simulink model "Integration_HILS_Filtered"  (R2023b)
settings: Solver=FixedStepAuto  StartTime=0.0  StopTime=inf  FixedStep=0.01  RelTol=1e-3  EnableMultiTasking=on
values from neighbouring files (symbols this model uses):
  batteryChargeRate = 0.0005    [paraHILS_File.m]
  batteryUpdateTime = 0.1    [paraHILS_File.m]
  batteryUseRate = 0.01    [paraHILS_File.m]
  encoder_scale = 1/12/4    (= 0.0208333333333)    [paraHILS_File.m]
  EncoderCutOffFreq = 48.1    [paraHILS_File.m]
  Ki = 10.0    (= 10)    [paraHILS_File.m]
  Kp = 10.0    (= 10)    [paraHILS_File.m]
  LimitMotorSpd = 0.8    [paraHILS_File.m]
  oilChargeRate = 2    [paraHILS_File.m]
  oilUpdateTime = 0.1    [paraHILS_File.m]
  oilUseRate = 0.01    [paraHILS_File.m]
  Vlim = 12    [paraHILS_File.m]
undefined symbols (not defined in the file or in its folder): MapVarRes2RPS
libraries: arduinolib x17, arduinosensorlib x2, simulink x2, cstblocks x2, dspstat3 x1
settings Model: ExtModeTrigDuration=2  Creator=sein  LastModifiedBy=hangbe
settings OptimizationCC: EnhancedBackFolding=on  PassReuseOutputArgsAs=Individual arguments  ZeroExternalMemoryAtStartup=off  ZeroInternalMemoryAtStartup=off  MaxStackSize=64  OptimizeBlockOrder=speed  DifferentSizesBufferReuse=on  OptimizationCustomize=off  EfficientTunableParamExpr=on
settings DebuggingCC: ParameterTunabilityLossMsg=error
settings HardwareCC: ProdBitPerInt=16  ProdBitPerPointer=16  ProdBitPerSizeT=16  ProdBitPerPtrDiffT=16  ProdLargestAtomicFloat=None  ProdWordSize=8  ProdHWDeviceType=Atmel->AVR
settings SFSimCC: MATLABDynamicMemAlloc=off
settings RTWCC: Description=Embedded Coder  SystemTargetFile=ert.tlc  HardwareBoard=Arduino Mega 2560  TemplateMakefile=ert_default_tmf  Toolchain=Arduino AVR  BuildConfiguration=Faster Runs
settings CodeAppCC: ForceParamTrailComments=on  IgnoreCustomStorageClasses=off  OperatorAnnotations=on  SimulinkDataObjDesc=on  SFDataObjDesc=on  InsertBlockDesc=on
settings ERTTargetCC: SupportContinuousTime=on  SupportVariableSizeSignals=on  ExtModeTransport=3  ExtModeStaticAlloc=on  ExtModeAutomaticAllocSize=off  ExtModeStaticAllocSize=2048  ExtModeMexFile=ext_xcp  ExtModeIntrfLevel=Level2 - Open

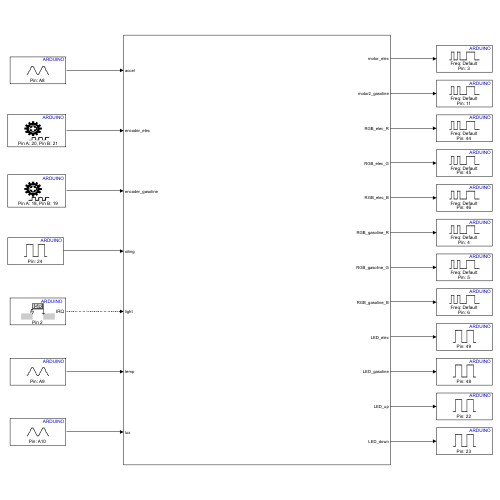
[thumbnail: Simulink's stored preview of the top-level diagram]
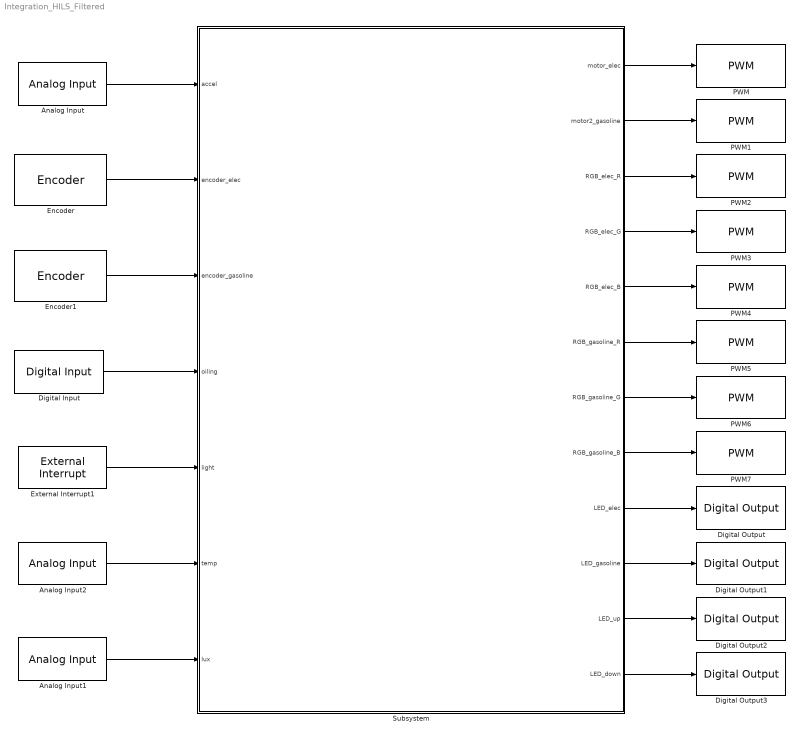
== system Integration_HILS_Filtered ==
  Analog Input : arduinolib/Analog Input  pinNumber=8  ReadResultsOnly=off  ConversionTriggerSource=Software  ExternalTriggerType=uint32( 0 )  OutputDataType=uint16  EnableConversionCompleteNotify=off  EnableOuputStatus=off  SampleTime=-1  blockPlatform=arduino
  Analog Input1 : arduinolib/Analog Input  pinNumber=10  ReadResultsOnly=off  ConversionTriggerSource=Software  ExternalTriggerType=uint32( 0 )  OutputDataType=uint16  EnableConversionCompleteNotify=off  EnableOuputStatus=off  SampleTime=-1  blockPlatform=arduino
  Analog Input2 : arduinolib/Analog Input  pinNumber=9  ReadResultsOnly=off  ConversionTriggerSource=Software  ExternalTriggerType=uint32( 0 )  OutputDataType=uint16  EnableConversionCompleteNotify=off  EnableOuputStatus=off  SampleTime=-1  blockPlatform=arduino
  Digital Input : arduinolib/Digital Input  pinNumber=24  mode=Default  Direction=input  SampleTime=0.1  blockPlatform=arduino
  Digital Output : arduinolib/Digital Output  pinNumber=49  Direction=output  blockPlatform=arduino
  Digital Output1 : arduinolib/Digital Output  pinNumber=48  Direction=output  blockPlatform=arduino
  Digital Output2 : arduinolib/Digital Output  pinNumber=22  Direction=output  blockPlatform=arduino
  Digital Output3 : arduinolib/Digital Output  pinNumber=23  Direction=output  blockPlatform=arduino
  Encoder : arduinosensorlib/Encoder  InputA=20  InputB=21  Mode=No reset  SampleTime=-1
  Encoder1 : arduinosensorlib/Encoder  InputA=18  InputB=19  Mode=No reset  SampleTime=-1
  External Interrupt1 : arduinolib/External Interrupt  Pin=2  PullUp=off  Mode=RISING  InterruptSimulationInput=off
  PWM : arduinolib/PWM  pinNumber=3  frequencyType=Default  desiredFrequency=490.2  achievableFrequency=490.2
  PWM1 : arduinolib/PWM  pinNumber=11  frequencyType=Default  desiredFrequency=490.2  achievableFrequency=490.2
  PWM2 : arduinolib/PWM  pinNumber=44  frequencyType=Default  desiredFrequency=490.2  achievableFrequency=490.2
  PWM3 : arduinolib/PWM  pinNumber=45  frequencyType=Default  desiredFrequency=490.2  achievableFrequency=490.2
  PWM4 : arduinolib/PWM  pinNumber=46  frequencyType=Default  desiredFrequency=490.2  achievableFrequency=490.2
  PWM5 : arduinolib/PWM  pinNumber=4  frequencyType=Default  desiredFrequency=490.2  achievableFrequency=490.2
  PWM6 : arduinolib/PWM  pinNumber=5  frequencyType=Default  desiredFrequency=490.2  achievableFrequency=490.2
  PWM7 : arduinolib/PWM  pinNumber=6  frequencyType=Default  desiredFrequency=490.2  achievableFrequency=490.2
  Subsystem : Subsystem
  wires:
  Analog Input/1 -> Subsystem/1(accel)
  Encoder/1 -> Subsystem/2(encoder_elec)
  Digital Input/1 -> Subsystem/4(oiling)
  External Interrupt1/1 -> Subsystem/5(light)
  Analog Input2/1 -> Subsystem/6(temp)
  Analog Input1/1 -> Subsystem/7(lux)
  Subsystem/1(motor_elec) -> PWM/1
  Subsystem/2(motor2_gasoline) -> PWM1/1
  Subsystem/3(RGB_elec_R) -> PWM2/1
  Subsystem/4(RGB_elec_G) -> PWM3/1
  Subsystem/5(RGB_elec_B) -> PWM4/1
  Subsystem/6(RGB_gasoline_R) -> PWM5/1
  Subsystem/7(RGB_gasoline_G) -> PWM6/1
  Subsystem/8(RGB_gasoline_B) -> PWM7/1
  Subsystem/9(LED_elec) -> Digital Output/1
  Subsystem/10(LED_gasoline) -> Digital Output1/1
  Subsystem/11(LED_up) -> Digital Output2/1
  Subsystem/12(LED_down) -> Digital Output3/1
  Encoder1/1 -> Subsystem/3(encoder_gasoline)

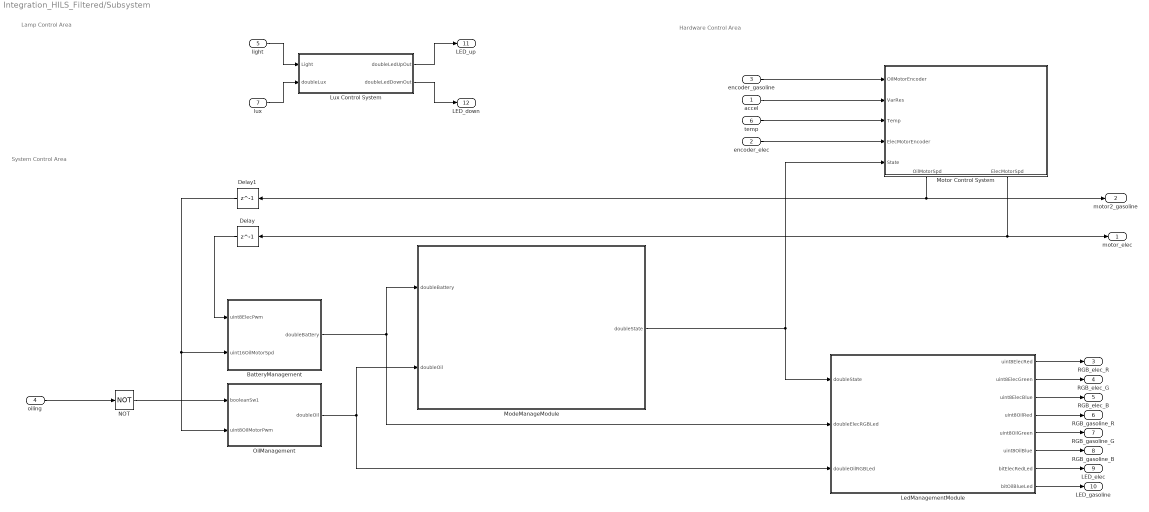
== system Integration_HILS_Filtered/Subsystem ==
  note: Lamp Control Area
  note: Hardware Control Area
  note: System Control Area
  accel : Inport
  encoder_elec : Inport  Port=2
  encoder_gasoline : Inport  Port=3
  oiling : Inport  Port=4
  light : Inport  Port=5
  temp : Inport  Port=6
  lux : Inport  Port=7
  BatteryManagement : Subsystem
  Delay : Delay  DelayLength=1
  Delay1 : Delay  DelayLength=1
  LedManagementModule : Subsystem
  Lux Control System : Subsystem
  ModeManageModule : Subsystem
  Motor Control System : Subsystem
      settings: PortSchema="{\"entries\":[{\"content\":{\"sides\":[{\"content\":{\"connectorIds\":[\"In1\",\"In2\",\"In3\",\"In4\",\"In5\"]},\"type\":\"ConnectorPlacement.EquallySpacedRectSide\",\"uuid\":\"d78dbdb5-4c64-485d-9b60-ddf3d4c9e050\"},{\"content\":{\"side\":\"RIGHT\"},\"type\":\"ConnectorPlacement.EquallySpacedRectSide\",\"uuid\":\"e4947276-b3db-4eab-ab89-2db109b5b76f\"},{\"content\":{\"side\":\"TOP\"},\"type\":\"ConnectorPlacement.EquallySpacedRectSide\",\"uuid\":\"f10de6be-2a9c-4a01-854d-c691ec39bdb2\"},{\"content\":{\"connectorIds\":[\"Out1\",\"Out2\"],\"side\":\"BOTTOM\"},\"type\":\"ConnectorPlacement.EquallySpacedRectSide\",\"uuid\":\"8b2dfeae-af3a-4cb1-8e5d-8c4928cafd33\"}]},\"type\":\"ConnectorPlacement.EquallySpacedConnector\",\"uuid\":\"966cd9e0-5a43-41a6-af76-62067303310a\"}],\"packageUris\":[\"http://schema.mathworks.com/mf0/Connector/R2020b\"],\"version\":\"1.0\"}"
  NOT : Logic  Operator=NOT  IconShape=distinctive  AllPortsSameDT=off  OutDataTypeStr=boolean
  OilManagement : Subsystem
  motor_elec : Outport
  motor2_gasoline : Outport  Port=2
  RGB_elec_R : Outport  Port=3
  RGB_elec_G : Outport  Port=4
  RGB_elec_B : Outport  Port=5
  RGB_gasoline_R : Outport  Port=6
  RGB_gasoline_G : Outport  Port=7
  RGB_gasoline_B : Outport  Port=8
  LED_elec : Outport  Port=9
  LED_gasoline : Outport  Port=10
  LED_up : Outport  Port=11
  LED_down : Outport  Port=12
  wires:
  LedManagementModule/1(uint8ElecRed) -> RGB_elec_R/1
  LedManagementModule/2(uint8ElecGreen) -> RGB_elec_G/1
  LedManagementModule/3(uint8ElecBlue) -> RGB_elec_B/1
  LedManagementModule/4(uint8OilRed) -> RGB_gasoline_R/1
  LedManagementModule/5(uint8OilGreen) -> RGB_gasoline_G/1
  LedManagementModule/6(uint8OilBlue) -> RGB_gasoline_B/1
  LedManagementModule/7(bitElecRedLed) -> LED_elec/1
  LedManagementModule/8(bitOilBlueLed) -> LED_gasoline/1
  ModeManageModule/1(doubleState) -> Motor Control System/5(State), LedManagementModule/1(doubleState)
  OilManagement/1(doubleOil) -> LedManagementModule/3(doubleOilRGBLed), ModeManageModule/2(doubleOil)
  oiling/1 -> NOT/1
  Delay/1 -> BatteryManagement/1(uint8ElecPwm)
  Delay1/1 -> OilManagement/2(uint8OilMotorPwm), BatteryManagement/2(uint16OilMotorSpd)
  NOT/1 -> OilManagement/1(booleanSw1)
  BatteryManagement/1(doubleBattery) -> LedManagementModule/2(doubleElecRGBLed), ModeManageModule/1(doubleBattery)
  light/1 -> Lux Control System/1(Light)
  lux/1 -> Lux Control System/2(doubleLux)
  Lux Control System/1(doubleLedUpOut) -> LED_up/1
  Lux Control System/2(doubleLedDownOut) -> LED_down/1
  Motor Control System/2(ElecMotorSpd) -> motor_elec/1, Delay/1
  Motor Control System/1(OilMotorSpd) -> motor2_gasoline/1, Delay1/1
  encoder_gasoline/1 -> Motor Control System/1(OilMotorEncoder)
  accel/1 -> Motor Control System/2(VarRes)
  temp/1 -> Motor Control System/3(Temp)
  encoder_elec/1 -> Motor Control System/4(ElecMotorEncoder)

== system Integration_HILS_Filtered/Subsystem/BatteryManagement ==
  uint8ElecPwm : Inport
  uint16OilMotorSpd : Inport  Port=2
  Chart : Stateflow chart  TreatAsAtomicUnit=on
  Data Type Conversion : DataTypeConversion  OutDataTypeStr=double  SaturateOnIntegerOverflow=off  RndMeth=Floor
  Data Type Conversion1 : DataTypeConversion  OutDataTypeStr=double  SaturateOnIntegerOverflow=off  RndMeth=Floor
  Display : Display
  doubleBattery : Outport  OutDataTypeStr=double
  wires:
  uint8ElecPwm/1 -> Data Type Conversion/1
  Chart/1(uint8Battery) -> doubleBattery/1, Display/1
  uint16OilMotorSpd/1 -> Data Type Conversion1/1
  Data Type Conversion/1 -> Chart/1(uint8ElecPwm)
  Data Type Conversion1/1 -> Chart/2(uint16OilMotorSpd)

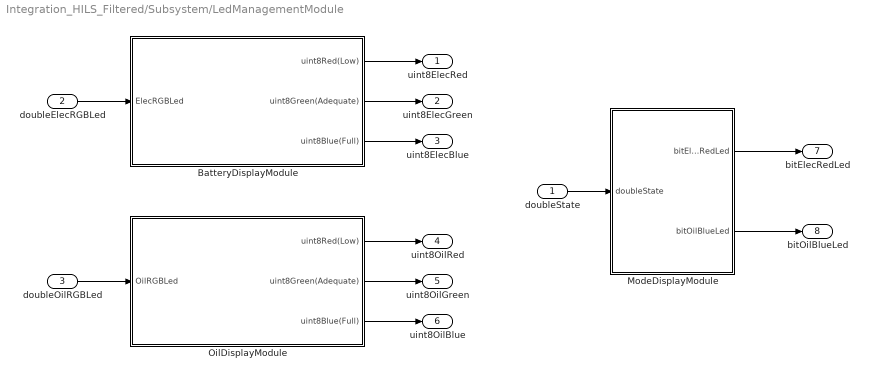
== system Integration_HILS_Filtered/Subsystem/LedManagementModule ==
  doubleState : Inport
  doubleElecRGBLed : Inport  Port=2
  doubleOilRGBLed : Inport  Port=3
  BatteryDisplayModule : Subsystem
  ModeDisplayModule : Subsystem
  OilDisplayModule : Subsystem
  uint8ElecRed : Outport
  uint8ElecGreen : Outport  Port=2
  uint8ElecBlue : Outport  Port=3
  uint8OilRed : Outport  Port=4
  uint8OilGreen : Outport  Port=5
  uint8OilBlue : Outport  Port=6
  bitElecRedLed : Outport  Port=7
  bitOilBlueLed : Outport  Port=8
  wires:
  OilDisplayModule/2(uint8Green(Adequate)) -> uint8OilGreen/1
  OilDisplayModule/3(uint8Blue(Full)) -> uint8OilBlue/1
  BatteryDisplayModule/1(uint8Red(Low)) -> uint8ElecRed/1
  BatteryDisplayModule/2(uint8Green(Adequate)) -> uint8ElecGreen/1
  OilDisplayModule/1(uint8Red(Low)) -> uint8OilRed/1
  BatteryDisplayModule/3(uint8Blue(Full)) -> uint8ElecBlue/1
  doubleOilRGBLed/1 -> OilDisplayModule/1(OilRGBLed)
  doubleElecRGBLed/1 -> BatteryDisplayModule/1(ElecRGBLed)
  doubleState/1 -> ModeDisplayModule/1(doubleState)
  ModeDisplayModule/2(bitOilBlueLed) -> bitOilBlueLed/1
  ModeDisplayModule/1(bitElecRedLed) -> bitElecRedLed/1

== system Integration_HILS_Filtered/Subsystem/Lux Control System ==
  Light : Inport
  doubleLux : Inport  Port=2
  LED_light_control : Subsystem
      settings: PortSchema="{\"entries\":[{\"content\":{\"sides\":[{\"content\":{\"connectorIds\":[\"In1\",\"In2\"]},\"type\":\"ConnectorPlacement.EquallySpacedRectSide\",\"uuid\":\"1bcc6ac7-15d7-4509-bf77-bbf32607b680\"},{\"content\":{\"connectorIds\":[\"Out1\",\"Out2\"],\"side\":\"RIGHT\"},\"type\":\"ConnectorPlacement.EquallySpacedRectSide\",\"uuid\":\"7c9447ca-d604-4256-8544-ba9898aaaccf\"},{\"content\":{\"connectorIds\":[\"In3\"],\"side\":\"TOP\"},\"type\":\"ConnectorPlacement.EquallySpacedRectSide\",\"uuid\":\"08491b94-2b66-4752-90e4-0e43207a446c\"}]},\"type\":\"ConnectorPlacement.EquallySpacedConnector\",\"uuid\":\"64a8cbb6-184c-45be-a1d8-1d8e5e745e8f\"}],\"packageUris\":[\"http://schema.mathworks.com/mf0/Connector/R2020b\"],\"version\":\"1.0\"}"
  lux_sensor : Subsystem
  sw_light : Subsystem
  doubleLedUpOut : Outport
  doubleLedDownOut : Outport  Port=2
  wires:
  doubleLux/1 -> lux_sensor/1(doubleLux)
  sw_light/1(doubleSwLight) -> LED_light_control/3(doubleSwLight)
  lux_sensor/1(doubleLedUp) -> LED_light_control/1(doubleLedUp)
  LED_light_control/2(doubleLedDownOut) -> doubleLedDownOut/1
  lux_sensor/2(doubleLedDown) -> LED_light_control/2(doubleLedDown)
  LED_light_control/1(doubleLedUpOut) -> doubleLedUpOut/1
  Light/1 -> sw_light/Trigger

== system Integration_HILS_Filtered/Subsystem/ModeManageModule ==
  doubleBattery : Inport
  doubleOil : Inport  Port=2
  Chart : Stateflow chart  TreatAsAtomicUnit=on
  doubleState : Outport
  wires:
  doubleBattery/1 -> Chart/1(Elec)
  doubleOil/1 -> Chart/2(Oil)
  Chart/1(State) -> doubleState/1

== system Integration_HILS_Filtered/Subsystem/Motor Control System ==
  OilMotorEncoder : Inport
  VarRes : Inport  Port=2
  Temp : Inport  Port=3
  ElecMotorEncoder : Inport  Port=4
  State : Inport  Port=5
  ElecMotorControl : Subsystem
  OilMotorControl1 : Subsystem
  OilMotorSpd : Outport
  ElecMotorSpd : Outport  Port=2
  wires:
  OilMotorControl1/1(OilMotorSpd) -> OilMotorSpd/1
  Temp/1 -> OilMotorControl1/3(Temp), ElecMotorControl/3(Temp)
  VarRes/1 -> OilMotorControl1/2(VarRes), ElecMotorControl/2(VarRes)
  ElecMotorEncoder/1 -> ElecMotorControl/4(ElecMotorEncoder)
  State/1 -> ElecMotorControl/1(State), OilMotorControl1/1(State)
  OilMotorEncoder/1 -> OilMotorControl1/4(OilMotorEncoder)
  ElecMotorControl/1(ElecMotorSpd) -> ElecMotorSpd/1

== system Integration_HILS_Filtered/Subsystem/OilManagement ==
  booleanSw1 : Inport
  uint8OilMotorPwm : Inport  Port=2
  Chart : Stateflow chart  TreatAsAtomicUnit=on
      settings: PortSchema="{\"entries\":[{\"content\":{\"sides\":[{\"content\":{\"connectorIds\":[\"In2\",\"In1\"]},\"type\":\"ConnectorPlacement.EquallySpacedRectSide\",\"uuid\":\"afc1c385-a15d-4992-a56e-13b091251b5d\"},{\"content\":{\"connectorIds\":[\"Out1\"],\"side\":\"RIGHT\"},\"type\":\"ConnectorPlacement.EquallySpacedRectSide\",\"uuid\":\"57c32afe-97af-4565-8322-9e1e1296b44d\"},{\"content\":{\"side\":\"TOP\"},\"type\":\"ConnectorPlacement.EquallySpacedRectSide\",\"uuid\":\"eea2667b-7f0f-4e05-8420-aa115f5842d9\"}]},\"type\":\"ConnectorPlacement.EquallySpacedConnector\",\"uuid\":\"005ff0fc-b81f-4bc1-a862-85c7c8646690\"}],\"packageUris\":[\"http://schema.mathworks.com/mf0/Connector/R2020b\"],\"version\":\"1.0\"}"
  Data Type Conversion : DataTypeConversion  OutDataTypeStr=double  SaturateOnIntegerOverflow=off  RndMeth=Floor
  Rate Transition : RateTransition
  doubleOil : Outport
  wires:
  Chart/1(doubleOil) -> doubleOil/1
  booleanSw1/1 -> Rate Transition/1
  uint8OilMotorPwm/1 -> Data Type Conversion/1
  Rate Transition/1 -> Chart/2(booleanSw1)
  Data Type Conversion/1 -> Chart/1(uint8OilMotorPwm)

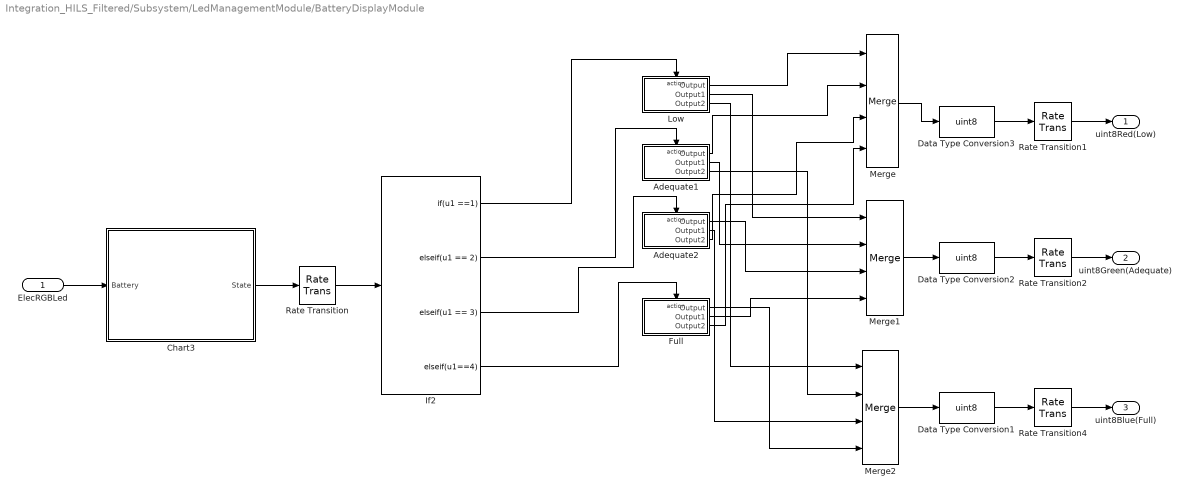
== system Integration_HILS_Filtered/Subsystem/LedManagementModule/BatteryDisplayModule ==
  ElecRGBLed : Inport
  Adequate1 : Subsystem  TreatAsAtomicUnit=on
  Adequate2 : Subsystem  TreatAsAtomicUnit=on
  Chart3 : Stateflow chart  TreatAsAtomicUnit=on
  Data Type Conversion1 : DataTypeConversion  OutDataTypeStr=uint8  SaturateOnIntegerOverflow=off  RndMeth=Floor
  Data Type Conversion2 : DataTypeConversion  OutDataTypeStr=uint8  SaturateOnIntegerOverflow=off  RndMeth=Floor
  Data Type Conversion3 : DataTypeConversion  OutDataTypeStr=uint8  SaturateOnIntegerOverflow=off  RndMeth=Floor
  Full : Subsystem  TreatAsAtomicUnit=on
  If2 : If  IfExpression=u1 ==1  ElseIfExpressions=u1 == 2, u1 == 3,u1==4  ShowElse=off
  Low : Subsystem  TreatAsAtomicUnit=on
  Merge : Merge  Inputs=4
  Merge1 : Merge  Inputs=4
  Merge2 : Merge  Inputs=4
  Rate Transition{,1..2,4} (4 alike) : RateTransition
  uint8Red(Low) : Outport
  uint8Green(Adequate) : Outport  Port=2
  uint8Blue(Full) : Outport  Port=3
  wires:
  Rate Transition/1 -> If2/1
  If2/1 -> Low/Action
  If2/2 -> Adequate1/Action
  Low/1(Output) -> Merge/1
  Adequate1/1(Output) -> Merge/2
  If2/3 -> Adequate2/Action
  If2/4 -> Full/Action
  Rate Transition4/1 -> uint8Blue(Full)/1
  Rate Transition1/1 -> uint8Red(Low)/1
  Merge1/1 -> Data Type Conversion2/1
  Merge2/1 -> Data Type Conversion1/1
  Data Type Conversion1/1 -> Rate Transition4/1
  Rate Transition2/1 -> uint8Green(Adequate)/1
  Data Type Conversion2/1 -> Rate Transition2/1
  Low/2(Output1) -> Merge1/1
  Low/3(Output2) -> Merge2/1
  Adequate1/2(Output1) -> Merge1/2
  Adequate1/3(Output2) -> Merge2/2
  Adequate2/1(Output) -> Merge1/3
  Adequate2/2(Output1) -> Merge2/3
  Full/1(Output) -> Merge2/4
  Full/2(Output1) -> Merge1/4
  ElecRGBLed/1 -> Chart3/1(Battery)
  Chart3/1(State) -> Rate Transition/1
  Merge/1 -> Data Type Conversion3/1
  Data Type Conversion3/1 -> Rate Transition1/1
  Adequate2/3(Output2) -> Merge/3
  Full/3(Output2) -> Merge/4

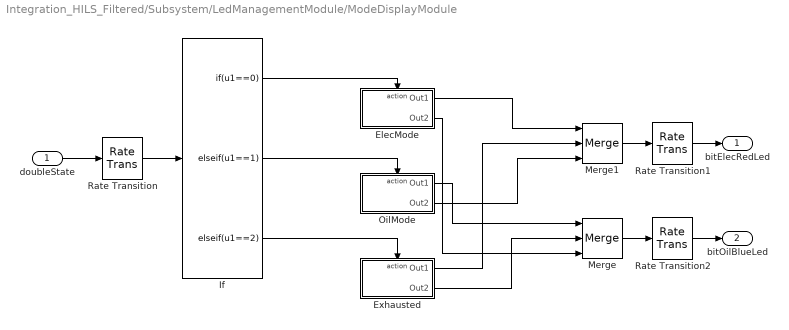
== system Integration_HILS_Filtered/Subsystem/LedManagementModule/ModeDisplayModule ==
  doubleState : Inport
  ElecMode : Subsystem  TreatAsAtomicUnit=on
  Exhausted : Subsystem  TreatAsAtomicUnit=on
  If : If  IfExpression=u1==0  ElseIfExpressions=u1==1, u1==2  ShowElse=off
  Merge : Merge  Inputs=3
  Merge1 : Merge  Inputs=3
  OilMode : Subsystem  TreatAsAtomicUnit=on
  Rate Transition : RateTransition
  Rate Transition1 : RateTransition
  Rate Transition2 : RateTransition
  bitElecRedLed : Outport
  bitOilBlueLed : Outport  Port=2
  wires:
  Exhausted/1(Out1) -> Merge1/2
  OilMode/1(Out1) -> Merge/1
  If/2 -> OilMode/Action
  OilMode/2(Out2) -> Merge1/3
  ElecMode/1(Out1) -> Merge1/1
  Exhausted/2(Out2) -> Merge/2
  If/3 -> Exhausted/Action
  If/1 -> ElecMode/Action
  ElecMode/2(Out2) -> Merge/3
  Rate Transition/1 -> If/1
  doubleState/1 -> Rate Transition/1
  Merge1/1 -> Rate Transition1/1
  Rate Transition1/1 -> bitElecRedLed/1
  Merge/1 -> Rate Transition2/1
  Rate Transition2/1 -> bitOilBlueLed/1

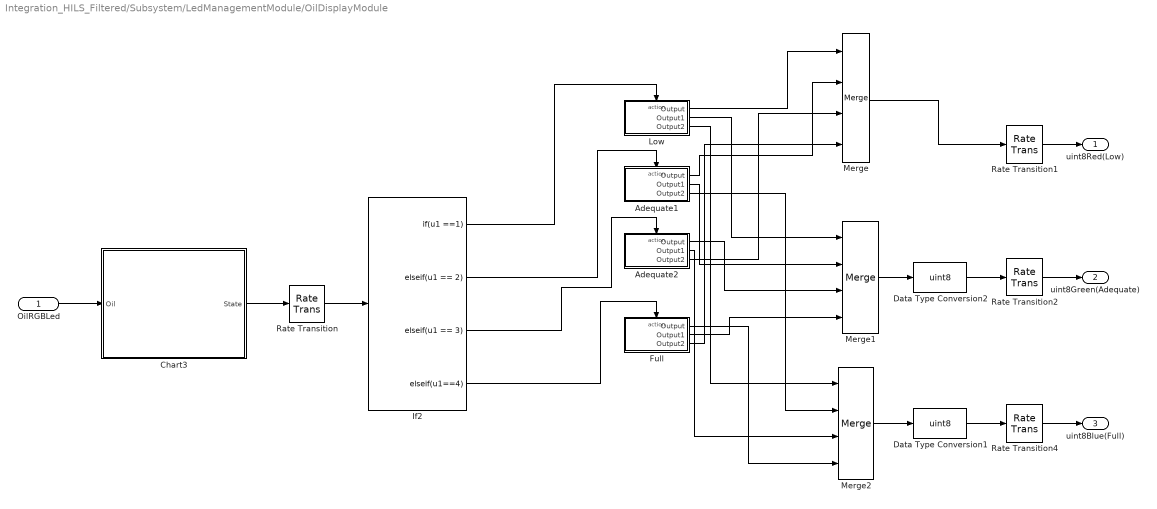
== system Integration_HILS_Filtered/Subsystem/LedManagementModule/OilDisplayModule ==
  OilRGBLed : Inport
  Adequate1 : Subsystem  TreatAsAtomicUnit=on
  Adequate2 : Subsystem  TreatAsAtomicUnit=on
  Chart3 : Stateflow chart  TreatAsAtomicUnit=on
  Data Type Conversion1 : DataTypeConversion  OutDataTypeStr=uint8  SaturateOnIntegerOverflow=off  RndMeth=Floor
  Data Type Conversion2 : DataTypeConversion  OutDataTypeStr=uint8  SaturateOnIntegerOverflow=off  RndMeth=Floor
  Full : Subsystem  TreatAsAtomicUnit=on
  If2 : If  IfExpression=u1 ==1  ElseIfExpressions=u1 == 2, u1 == 3,u1==4  ShowElse=off
  Low : Subsystem  TreatAsAtomicUnit=on
  Merge : Merge  Inputs=4
  Merge1 : Merge  Inputs=4
  Merge2 : Merge  Inputs=4
  Rate Transition{,1..2,4} (4 alike) : RateTransition
  uint8Red(Low) : Outport
  uint8Green(Adequate) : Outport  Port=2
  uint8Blue(Full) : Outport  Port=3
  wires:
  Chart3/1(State) -> Rate Transition/1
  OilRGBLed/1 -> Chart3/1(Oil)
  Full/2(Output1) -> Merge1/4
  Full/1(Output) -> Merge2/4
  Adequate2/2(Output1) -> Merge2/3
  Adequate2/1(Output) -> Merge1/3
  Adequate1/3(Output2) -> Merge2/2
  Adequate1/2(Output1) -> Merge1/2
  Low/3(Output2) -> Merge2/1
  Low/2(Output1) -> Merge1/1
  Data Type Conversion2/1 -> Rate Transition2/1
  Rate Transition2/1 -> uint8Green(Adequate)/1
  Data Type Conversion1/1 -> Rate Transition4/1
  Merge2/1 -> Data Type Conversion1/1
  Merge1/1 -> Data Type Conversion2/1
  Rate Transition1/1 -> uint8Red(Low)/1
  Merge/1 -> Rate Transition1/1
  Rate Transition4/1 -> uint8Blue(Full)/1
  If2/4 -> Full/Action
  If2/3 -> Adequate2/Action
  Adequate1/1(Output) -> Merge/2
  Low/1(Output) -> Merge/1
  If2/2 -> Adequate1/Action
  If2/1 -> Low/Action
  Rate Transition/1 -> If2/1
  Adequate2/3(Output2) -> Merge/3
  Full/3(Output2) -> Merge/4

== system Integration_HILS_Filtered/Subsystem/Lux Control System/LED_light_control ==
  doubleLedUp : Inport
  doubleLedDown : Inport  Port=2
  doubleSwLight : Inport  Port=3
  Product : Product
  Product1 : Product
  Rate Transition : RateTransition  Integrity=off
  doubleLedUpOut : Outport
  doubleLedDownOut : Outport  Port=2
  wires:
  Rate Transition/1 -> Product1/1, Product/2
  Product1/1 -> doubleLedDownOut/1
  Product/1 -> doubleLedUpOut/1
  doubleSwLight/1 -> Rate Transition/1
  doubleLedUp/1 -> Product/1
  doubleLedDown/1 -> Product1/2

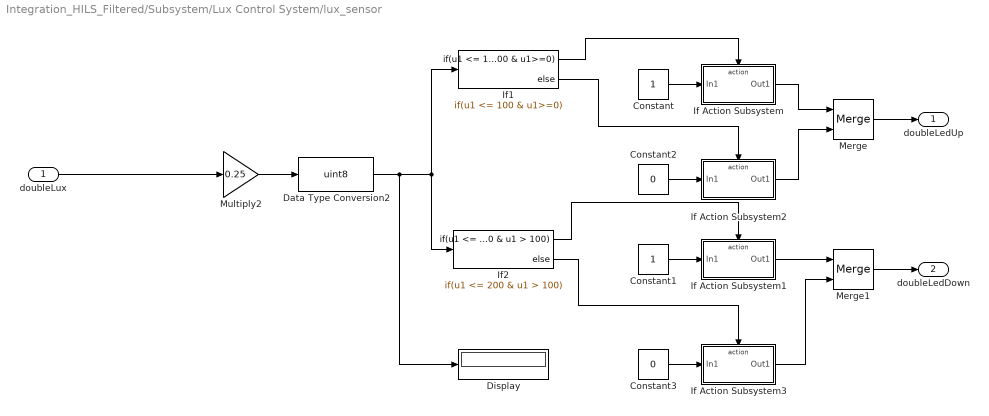
== system Integration_HILS_Filtered/Subsystem/Lux Control System/lux_sensor ==
  doubleLux : Inport
  Constant : Constant
  Constant1 : Constant
  Constant2 : Constant  Value=0
  Constant3 : Constant  Value=0
  Data Type Conversion2 : DataTypeConversion  OutDataTypeStr=uint8  SaturateOnIntegerOverflow=off  RndMeth=Floor
  Display : Display
  If Action Subsystem : Subsystem  TreatAsAtomicUnit=on
  If Action Subsystem1 : Subsystem  TreatAsAtomicUnit=on
  If Action Subsystem2 : Subsystem  TreatAsAtomicUnit=on
  If Action Subsystem3 : Subsystem  TreatAsAtomicUnit=on
  If1 : If  IfExpression=u1 <= 100 & u1>=0
  If2 : If  IfExpression=u1 <= 200 & u1 > 100
  Merge : Merge
  Merge1 : Merge
  Multiply2 : Gain  Gain=0.25
  doubleLedUp : Outport
  doubleLedDown : Outport  Port=2
  wires:
  If1/2 -> If Action Subsystem2/Action
  If2/2 -> If Action Subsystem3/Action
  Constant2/1 -> If Action Subsystem2/1(In1)
  Merge/1 -> doubleLedUp/1
  If Action Subsystem2/1(Out1) -> Merge/2
  Multiply2/1 -> Data Type Conversion2/1
  Constant/1 -> If Action Subsystem/1(In1)
  If2/1 -> If Action Subsystem1/Action
  If1/1 -> If Action Subsystem/Action
  Constant1/1 -> If Action Subsystem1/1(In1)
  doubleLux/1 -> Multiply2/1
  Constant3/1 -> If Action Subsystem3/1(In1)
  Merge1/1 -> doubleLedDown/1
  If Action Subsystem/1(Out1) -> Merge/1
  If Action Subsystem1/1(Out1) -> Merge1/1
  Data Type Conversion2/1 -> If1/1, If2/1, Display/1
  If Action Subsystem3/1(Out1) -> Merge1/2

== system Integration_HILS_Filtered/Subsystem/Lux Control System/sw_light ==
  function : TriggerPort  TriggerType=function-call  VariantControl=(inherit)
  Delay2 : Delay  DelayLength=1
  NOT : Logic  Operator=NOT  IconShape=distinctive  AllPortsSameDT=off  OutDataTypeStr=boolean
  doubleSwLight : Outport
  wires:
  NOT/1 -> doubleSwLight/1, Delay2/1
  Delay2/1 -> NOT/1

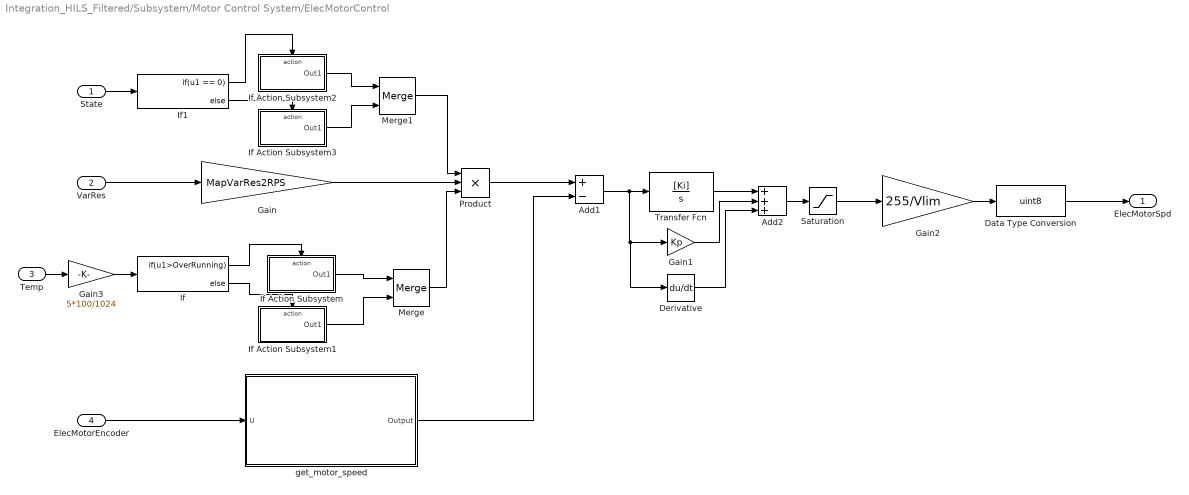
== system Integration_HILS_Filtered/Subsystem/Motor Control System/ElecMotorControl ==
  State : Inport
  VarRes : Inport  Port=2
  Temp : Inport  Port=3
  ElecMotorEncoder : Inport  Port=4
  Add1 : Sum  Inputs=+-
  Add2 : Sum  Inputs=+++
  Data Type Conversion : DataTypeConversion  OutDataTypeStr=uint8  SaturateOnIntegerOverflow=off  RndMeth=Floor
  Derivative : Derivative  CoefficientInTFapproximation=Kd
  Gain : Gain  Gain=MapVarRes2RPS
  Gain1 : Gain  Gain=Kp
  Gain2 : Gain  Gain=255/Vlim
  Gain3 : Gain  Gain=5*100/1024  ParamDataTypeStr=double
  If : If  IfExpression=u1>OverRunning
  If Action Subsystem : Subsystem  TreatAsAtomicUnit=on
  If Action Subsystem1 : Subsystem  TreatAsAtomicUnit=on
  If Action Subsystem2 : Subsystem  TreatAsAtomicUnit=on
  If Action Subsystem3 : Subsystem  TreatAsAtomicUnit=on
  If1 : If  IfExpression=u1 == 0
  Merge : Merge
  Merge1 : Merge
  Product : Product  Inputs=3
  Saturation : Saturate  UpperLimit=Vlim  LowerLimit=0
  Transfer Fcn : TransferFcn  Numerator=[Ki]  Denominator=[1 0]
  get_motor_speed : Subsystem
  ElecMotorSpd : Outport
  wires:
  If/2 -> If Action Subsystem1/Action
  Transfer Fcn/1 -> Add2/1
  Add1/1 -> Derivative/1, Gain1/1, Transfer Fcn/1
  Data Type Conversion/1 -> ElecMotorSpd/1
  Add2/1 -> Saturation/1
  If/1 -> If Action Subsystem/Action
  Saturation/1 -> Gain2/1
  Gain1/1 -> Add2/2
  Merge/1 -> Product/3
  If Action Subsystem1/1(Out1) -> Merge/2
  Derivative/1 -> Add2/3
  Product/1 -> Add1/1
  If Action Subsystem/1(Out1) -> Merge/1
  Temp/1 -> Gain3/1
  State/1 -> If1/1
  If1/1 -> If Action Subsystem2/Action
  If1/2 -> If Action Subsystem3/Action
  If Action Subsystem2/1(Out1) -> Merge1/1
  If Action Subsystem3/1(Out1) -> Merge1/2
  Merge1/1 -> Product/1
  VarRes/1 -> Gain/1
  Gain/1 -> Product/2
  ElecMotorEncoder/1 -> get_motor_speed/1(U)
  get_motor_speed/1(Output) -> Add1/2
  Gain2/1 -> Data Type Conversion/1
  Gain3/1 -> If/1

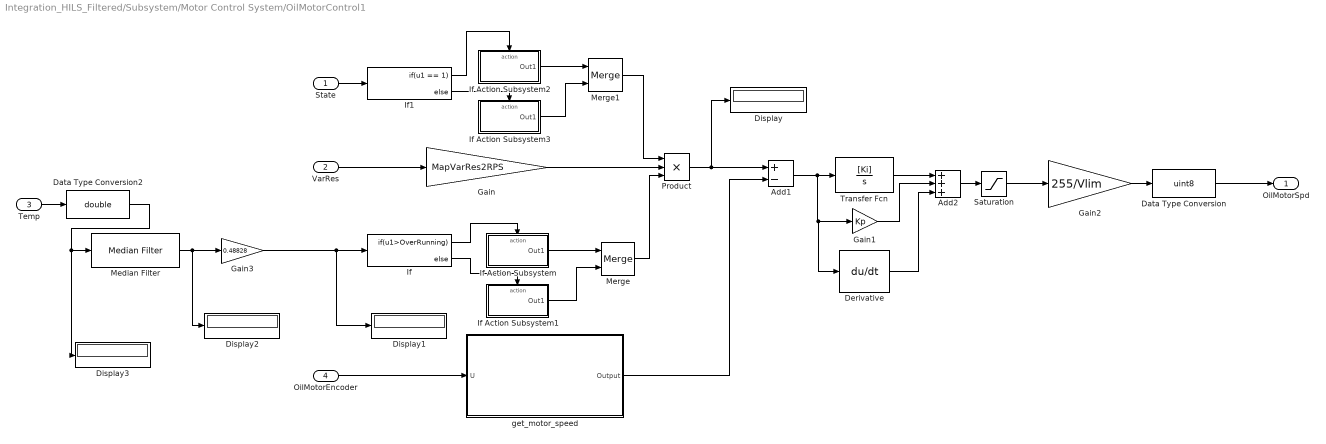
== system Integration_HILS_Filtered/Subsystem/Motor Control System/OilMotorControl1 ==
  State : Inport
  VarRes : Inport  Port=2
  Temp : Inport  Port=3
  OilMotorEncoder : Inport  Port=4
  Add1 : Sum  Inputs=+-
  Add2 : Sum  Inputs=+++
  Data Type Conversion : DataTypeConversion  OutDataTypeStr=uint8  SaturateOnIntegerOverflow=off  RndMeth=Floor
  Data Type Conversion2 : DataTypeConversion  OutDataTypeStr=double  SaturateOnIntegerOverflow=off  RndMeth=Floor
  Derivative : Derivative  CoefficientInTFapproximation=Kd
  Display{,1..3} (4 alike) : Display
  Gain : Gain  Gain=MapVarRes2RPS
  Gain1 : Gain  Gain=Kp
  Gain2 : Gain  Gain=255/Vlim
  Gain3 : Gain  Gain=0.48828  ParamDataTypeStr=double  OutDataTypeStr=double
  If : If  IfExpression=u1>OverRunning
  If Action Subsystem : Subsystem  TreatAsAtomicUnit=on
  If Action Subsystem1 : Subsystem  TreatAsAtomicUnit=on
  If Action Subsystem2 : Subsystem  TreatAsAtomicUnit=on
  If Action Subsystem3 : Subsystem  TreatAsAtomicUnit=on
  If1 : If  IfExpression=u1 == 1
  Median Filter : dspstat3/Median Filter  WindowLength=5  SimulateUsing=Interpreted execution
      settings: LibrarySourceBlock=|
      | dspfdesign/Median
      | Filter
  Merge : Merge
  Merge1 : Merge
  Product : Product  Inputs=3
  Saturation : Saturate  UpperLimit=Vlim  LowerLimit=0
  Transfer Fcn : TransferFcn  Numerator=[Ki]  Denominator=[1 0]
  get_motor_speed : Subsystem
  OilMotorSpd : Outport
  wires:
  If/2 -> If Action Subsystem1/Action
  Transfer Fcn/1 -> Add2/1
  Add1/1 -> Derivative/1, Gain1/1, Transfer Fcn/1
  Data Type Conversion/1 -> OilMotorSpd/1
  Add2/1 -> Saturation/1
  If/1 -> If Action Subsystem/Action
  Saturation/1 -> Gain2/1
  Gain1/1 -> Add2/2
  Merge/1 -> Product/3
  If Action Subsystem1/1(Out1) -> Merge/2
  Derivative/1 -> Add2/3
  If Action Subsystem/1(Out1) -> Merge/1
  State/1 -> If1/1
  If1/1 -> If Action Subsystem2/Action
  If1/2 -> If Action Subsystem3/Action
  If Action Subsystem2/1(Out1) -> Merge1/1
  If Action Subsystem3/1(Out1) -> Merge1/2
  Merge1/1 -> Product/1
  VarRes/1 -> Gain/1
  Gain/1 -> Product/2
  OilMotorEncoder/1 -> get_motor_speed/1(U)
  Gain2/1 -> Data Type Conversion/1
  get_motor_speed/1(Output) -> Add1/2
  Product/1 -> Display/1, Add1/1
  Gain3/1 -> Display1/1, If/1
  Median Filter/1 -> Display2/1, Gain3/1
  Temp/1 -> Data Type Conversion2/1
  Data Type Conversion2/1 -> Display3/1, Median Filter/1

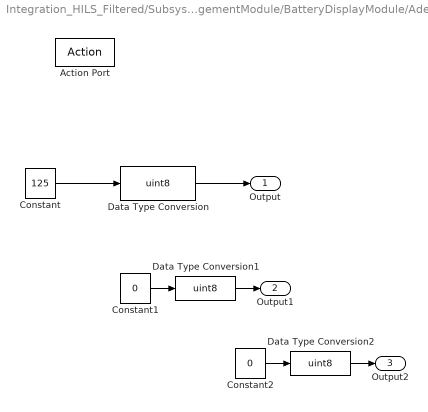
== system Integration_HILS_Filtered/Subsystem/LedManagementModule/BatteryDisplayModule/Adequate1 ==
  Action Port : ActionPort  ActionPortLabel=elseif(u1 == 2)
  Constant : Constant  Value=125
  Constant1 : Constant  Value=0
  Constant2 : Constant  Value=0
  Data Type Conversion : DataTypeConversion  OutDataTypeStr=uint8  SaturateOnIntegerOverflow=off  RndMeth=Floor
  Data Type Conversion1 : DataTypeConversion  OutDataTypeStr=uint8  SaturateOnIntegerOverflow=off  RndMeth=Floor
  Data Type Conversion2 : DataTypeConversion  OutDataTypeStr=uint8  SaturateOnIntegerOverflow=off  RndMeth=Floor
  Output : Outport
  Output1 : Outport  Port=2
  Output2 : Outport  Port=3
  wires:
  Data Type Conversion/1 -> Output/1
  Constant/1 -> Data Type Conversion/1
  Constant1/1 -> Data Type Conversion1/1
  Data Type Conversion1/1 -> Output1/1
  Constant2/1 -> Data Type Conversion2/1
  Data Type Conversion2/1 -> Output2/1

== system Integration_HILS_Filtered/Subsystem/LedManagementModule/BatteryDisplayModule/Adequate2 ==
  Action Port : ActionPort  ActionPortLabel=elseif( u1 == 3)
  Constant : Constant  Value=125
  Constant1 : Constant  Value=0
  Constant2 : Constant  Value=0
  Data Type Conversion : DataTypeConversion  OutDataTypeStr=uint8  SaturateOnIntegerOverflow=off  RndMeth=Floor
  Data Type Conversion1 : DataTypeConversion  OutDataTypeStr=uint8  SaturateOnIntegerOverflow=off  RndMeth=Floor
  Data Type Conversion2 : DataTypeConversion  OutDataTypeStr=uint8  SaturateOnIntegerOverflow=off  RndMeth=Floor
  Output : Outport
  Output1 : Outport  Port=2
  Output2 : Outport  Port=3
  wires:
  Data Type Conversion/1 -> Output/1
  Constant/1 -> Data Type Conversion/1
  Constant1/1 -> Data Type Conversion1/1
  Data Type Conversion1/1 -> Output1/1
  Data Type Conversion2/1 -> Output2/1
  Constant2/1 -> Data Type Conversion2/1

== system Integration_HILS_Filtered/Subsystem/LedManagementModule/BatteryDisplayModule/Full ==
  Action Port : ActionPort  ActionPortLabel=elseif(u1==4)
  Constant : Constant  Value=125
  Constant1 : Constant  Value=0
  Constant2 : Constant  Value=0
  Data Type Conversion : DataTypeConversion  OutDataTypeStr=uint8  SaturateOnIntegerOverflow=off  RndMeth=Floor
  Data Type Conversion1 : DataTypeConversion  OutDataTypeStr=uint8  SaturateOnIntegerOverflow=off  RndMeth=Floor
  Data Type Conversion2 : DataTypeConversion  OutDataTypeStr=uint8  SaturateOnIntegerOverflow=off  RndMeth=Floor
  Output : Outport
  Output1 : Outport  Port=2
  Output2 : Outport  Port=3
  wires:
  Constant/1 -> Data Type Conversion/1
  Data Type Conversion/1 -> Output/1
  Constant1/1 -> Data Type Conversion1/1
  Data Type Conversion1/1 -> Output1/1
  Data Type Conversion2/1 -> Output2/1
  Constant2/1 -> Data Type Conversion2/1

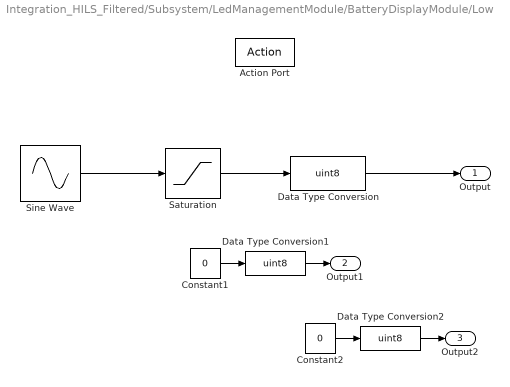
== system Integration_HILS_Filtered/Subsystem/LedManagementModule/BatteryDisplayModule/Low ==
  Action Port : ActionPort  ActionPortLabel=if(u1 ==1)
  Constant1 : Constant  Value=0
  Constant2 : Constant  Value=0
  Data Type Conversion : DataTypeConversion  OutDataTypeStr=uint8  SaturateOnIntegerOverflow=off  RndMeth=Floor
  Data Type Conversion1 : DataTypeConversion  OutDataTypeStr=uint8  SaturateOnIntegerOverflow=off  RndMeth=Floor
  Data Type Conversion2 : DataTypeConversion  OutDataTypeStr=uint8  SaturateOnIntegerOverflow=off  RndMeth=Floor
  Saturation : Saturate  UpperLimit=100  LowerLimit=0
  Sine Wave : Sin  Amplitude=100  Frequency=2*pi*3  SampleTime=0
  Output : Outport
  Output1 : Outport  Port=2
  Output2 : Outport  Port=3
  wires:
  Sine Wave/1 -> Saturation/1
  Saturation/1 -> Data Type Conversion/1
  Data Type Conversion/1 -> Output/1
  Constant1/1 -> Data Type Conversion1/1
  Data Type Conversion1/1 -> Output1/1
  Data Type Conversion2/1 -> Output2/1
  Constant2/1 -> Data Type Conversion2/1

== system Integration_HILS_Filtered/Subsystem/LedManagementModule/ModeDisplayModule/ElecMode ==
  Action Port : ActionPort  ActionPortLabel=if(u1==0)
  Constant1 : Constant  Value=0
  Pulse Generator : DiscretePulseGenerator  PulseType=Time based  PulseWidth=50
  Out1 : Outport
  Out2 : Outport  Port=2
  wires:
  Constant1/1 -> Out2/1
  Pulse Generator/1 -> Out1/1

== system Integration_HILS_Filtered/Subsystem/LedManagementModule/ModeDisplayModule/Exhausted ==
  Action Port : ActionPort  ActionPortLabel=elseif( u1==2)
  Constant : Constant  Value=0
  Constant1 : Constant  Value=0
  Out1 : Outport
  Out2 : Outport  Port=2
  wires:
  Constant/1 -> Out1/1
  Constant1/1 -> Out2/1

== system Integration_HILS_Filtered/Subsystem/LedManagementModule/ModeDisplayModule/OilMode ==
  Action Port : ActionPort  ActionPortLabel=elseif(u1==1)
  Constant : Constant  Value=0
  Pulse Generator : DiscretePulseGenerator  PulseType=Time based  PulseWidth=50
  Out1 : Outport
  Out2 : Outport  Port=2
  wires:
  Pulse Generator/1 -> Out1/1
  Constant/1 -> Out2/1

== system Integration_HILS_Filtered/Subsystem/LedManagementModule/OilDisplayModule/Adequate1 ==
  Action Port : ActionPort  ActionPortLabel=elseif(u1 == 2)
  Constant : Constant  Value=125
  Constant1 : Constant  Value=0
  Constant2 : Constant  Value=0
  Data Type Conversion : DataTypeConversion  OutDataTypeStr=uint8  SaturateOnIntegerOverflow=off  RndMeth=Floor
  Data Type Conversion1 : DataTypeConversion  OutDataTypeStr=uint8  SaturateOnIntegerOverflow=off  RndMeth=Floor
  Data Type Conversion2 : DataTypeConversion  OutDataTypeStr=uint8  SaturateOnIntegerOverflow=off  RndMeth=Floor
  Output : Outport
  Output1 : Outport  Port=2
  Output2 : Outport  Port=3
  wires:
  Data Type Conversion2/1 -> Output2/1
  Constant2/1 -> Data Type Conversion2/1
  Data Type Conversion1/1 -> Output1/1
  Constant1/1 -> Data Type Conversion1/1
  Constant/1 -> Data Type Conversion/1
  Data Type Conversion/1 -> Output/1

== system Integration_HILS_Filtered/Subsystem/LedManagementModule/OilDisplayModule/Adequate2 ==
  Action Port : ActionPort  ActionPortLabel=elseif( u1 == 3)
  Constant : Constant  Value=125
  Constant1 : Constant  Value=0
  Constant2 : Constant  Value=0
  Data Type Conversion : DataTypeConversion  OutDataTypeStr=uint8  SaturateOnIntegerOverflow=off  RndMeth=Floor
  Data Type Conversion1 : DataTypeConversion  OutDataTypeStr=uint8  SaturateOnIntegerOverflow=off  RndMeth=Floor
  Data Type Conversion2 : DataTypeConversion  OutDataTypeStr=uint8  SaturateOnIntegerOverflow=off  RndMeth=Floor
  Output : Outport
  Output1 : Outport  Port=2
  Output2 : Outport  Port=3
  wires:
  Data Type Conversion1/1 -> Output1/1
  Constant1/1 -> Data Type Conversion1/1
  Constant/1 -> Data Type Conversion/1
  Data Type Conversion/1 -> Output/1
  Data Type Conversion2/1 -> Output2/1
  Constant2/1 -> Data Type Conversion2/1

== system Integration_HILS_Filtered/Subsystem/LedManagementModule/OilDisplayModule/Full ==
  Action Port : ActionPort  ActionPortLabel=elseif(u1==4)
  Constant : Constant  Value=125
  Constant1 : Constant  Value=0
  Constant2 : Constant  Value=0
  Data Type Conversion : DataTypeConversion  OutDataTypeStr=uint8  SaturateOnIntegerOverflow=off  RndMeth=Floor
  Data Type Conversion1 : DataTypeConversion  OutDataTypeStr=uint8  SaturateOnIntegerOverflow=off  RndMeth=Floor
  Data Type Conversion2 : DataTypeConversion  OutDataTypeStr=uint8  SaturateOnIntegerOverflow=off  RndMeth=Floor
  Output : Outport
  Output1 : Outport  Port=2
  Output2 : Outport  Port=3
  wires:
  Data Type Conversion1/1 -> Output1/1
  Constant1/1 -> Data Type Conversion1/1
  Data Type Conversion/1 -> Output/1
  Constant/1 -> Data Type Conversion/1
  Data Type Conversion2/1 -> Output2/1
  Constant2/1 -> Data Type Conversion2/1

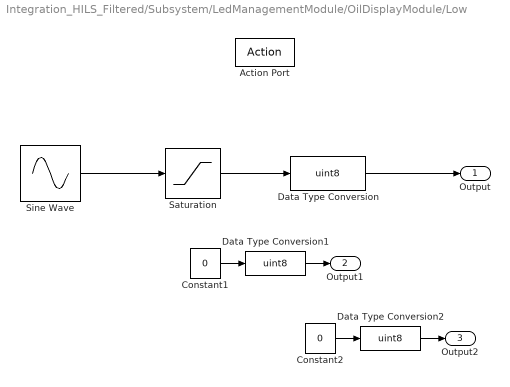
== system Integration_HILS_Filtered/Subsystem/LedManagementModule/OilDisplayModule/Low ==
  Action Port : ActionPort  ActionPortLabel=if(u1 ==1)
  Constant1 : Constant  Value=0
  Constant2 : Constant  Value=0
  Data Type Conversion : DataTypeConversion  OutDataTypeStr=uint8  SaturateOnIntegerOverflow=off  RndMeth=Floor
  Data Type Conversion1 : DataTypeConversion  OutDataTypeStr=uint8  SaturateOnIntegerOverflow=off  RndMeth=Floor
  Data Type Conversion2 : DataTypeConversion  OutDataTypeStr=uint8  SaturateOnIntegerOverflow=off  RndMeth=Floor
  Saturation : Saturate  UpperLimit=100  LowerLimit=0
  Sine Wave : Sin  Amplitude=100  Frequency=2*pi*3  SampleTime=0
  Output : Outport
  Output1 : Outport  Port=2
  Output2 : Outport  Port=3
  wires:
  Constant2/1 -> Data Type Conversion2/1
  Data Type Conversion2/1 -> Output2/1
  Data Type Conversion1/1 -> Output1/1
  Constant1/1 -> Data Type Conversion1/1
  Data Type Conversion/1 -> Output/1
  Saturation/1 -> Data Type Conversion/1
  Sine Wave/1 -> Saturation/1

== system Integration_HILS_Filtered/Subsystem/Lux Control System/lux_sensor/If Action Subsystem ==
  In1 : Inport
  Action Port : ActionPort  ActionPortLabel=if(u1 <= 100 & u1>=0)
  Out1 : Outport
  wires:
  In1/1 -> Out1/1

== system Integration_HILS_Filtered/Subsystem/Lux Control System/lux_sensor/If Action Subsystem1 ==
  In1 : Inport
  Action Port : ActionPort  ActionPortLabel=if(u1 <= 200 & u1 > 100)
  Out1 : Outport
  wires:
  In1/1 -> Out1/1

== system Integration_HILS_Filtered/Subsystem/Lux Control System/lux_sensor/If Action Subsystem2 ==
  In1 : Inport
  Action Port : ActionPort  ActionPortLabel=else
  Out1 : Outport
  wires:
  In1/1 -> Out1/1

== system Integration_HILS_Filtered/Subsystem/Lux Control System/lux_sensor/If Action Subsystem3 ==
  In1 : Inport
  Action Port : ActionPort  ActionPortLabel=else
  Out1 : Outport
  wires:
  In1/1 -> Out1/1

== system Integration_HILS_Filtered/Subsystem/Motor Control System/ElecMotorControl/If Action Subsystem ==
  Action Port : ActionPort  ActionPortLabel=if(u1>OverRunning)
  Constant : Constant  Value=LimitMotorSpd
  Out1 : Outport
  wires:
  Constant/1 -> Out1/1

== system Integration_HILS_Filtered/Subsystem/Motor Control System/ElecMotorControl/If Action Subsystem1 ==
  Action Port : ActionPort  ActionPortLabel=else
  Constant : Constant
  Out1 : Outport
  wires:
  Constant/1 -> Out1/1

== system Integration_HILS_Filtered/Subsystem/Motor Control System/ElecMotorControl/If Action Subsystem2 ==
  Action Port : ActionPort  ActionPortLabel=if(u1 == 0)
  Constant : Constant
  Out1 : Outport
  wires:
  Constant/1 -> Out1/1

== system Integration_HILS_Filtered/Subsystem/Motor Control System/ElecMotorControl/If Action Subsystem3 ==
  Action Port : ActionPort  ActionPortLabel=else
  Constant : Constant  Value=0
  Out1 : Outport
  wires:
  Constant/1 -> Out1/1

== system Integration_HILS_Filtered/Subsystem/Motor Control System/ElecMotorControl/get_motor_speed ==
  U : Inport
  Data Type Conversion : DataTypeConversion  OutDataTypeStr=int32  SaturateOnIntegerOverflow=off  RndMeth=Floor
  Discrete Derivative : simulink/Discrete/Discrete Derivative  gainval=1.0  ICPrevScaledInput=0.0  OutMin=[]  OutMax=[]  OutDataType=fixdt(1, 16)  OutScaling=2^-10  DoSatur=off
  EncoderCutOffFreq : Constant  Value=EncoderCutOffFreq
  Gain : Gain  Gain=encoder_scale
  Scope : Scope
  Varying Lowpass Filter : cstblocks/Linear Parameter Varying/Varying Lowpass Filter  N=1
  Output : Outport
  wires:
  Gain/1 -> Data Type Conversion/1
  U/1 -> Discrete Derivative/1, Scope/1
  Data Type Conversion/1 -> Output/1
  Varying Lowpass Filter/1 -> Gain/1
  Discrete Derivative/1 -> Varying Lowpass Filter/1
  EncoderCutOffFreq/1 -> Varying Lowpass Filter/2

== system Integration_HILS_Filtered/Subsystem/Motor Control System/OilMotorControl1/If Action Subsystem ==
  Action Port : ActionPort  ActionPortLabel=if(u1>OverRunning)
  Constant : Constant  Value=LimitMotorSpd
  Out1 : Outport
  wires:
  Constant/1 -> Out1/1

== system Integration_HILS_Filtered/Subsystem/Motor Control System/OilMotorControl1/If Action Subsystem1 ==
  Action Port : ActionPort  ActionPortLabel=else
  Constant : Constant
  Out1 : Outport
  wires:
  Constant/1 -> Out1/1

== system Integration_HILS_Filtered/Subsystem/Motor Control System/OilMotorControl1/If Action Subsystem2 ==
  Action Port : ActionPort  ActionPortLabel=if(u1 == 1)
  Constant : Constant
  Out1 : Outport
  wires:
  Constant/1 -> Out1/1

== system Integration_HILS_Filtered/Subsystem/Motor Control System/OilMotorControl1/If Action Subsystem3 ==
  Action Port : ActionPort  ActionPortLabel=else
  Constant : Constant  Value=0
  Out1 : Outport
  wires:
  Constant/1 -> Out1/1

== system Integration_HILS_Filtered/Subsystem/Motor Control System/OilMotorControl1/get_motor_speed ==
  U : Inport
  CutOffFreqeuncy : Constant  Value=EncoderCutOffFreq
  Data Type Conversion : DataTypeConversion  OutDataTypeStr=int32  SaturateOnIntegerOverflow=off  RndMeth=Floor
  Discrete Derivative : simulink/Discrete/Discrete Derivative  gainval=1.0  ICPrevScaledInput=0.0  OutMin=[]  OutMax=[]  OutDataType=fixdt(1, 16)  OutScaling=2^-10  DoSatur=off
  Gain : Gain  Gain=encoder_scale
  Scope : Scope
  Varying Lowpass Filter : cstblocks/Linear Parameter Varying/Varying Lowpass Filter  N=1
  Output : Outport
  wires:
  Gain/1 -> Data Type Conversion/1
  U/1 -> Discrete Derivative/1, Scope/1
  Data Type Conversion/1 -> Output/1
  Discrete Derivative/1 -> Varying Lowpass Filter/1
  Varying Lowpass Filter/1 -> Gain/1
  CutOffFreqeuncy/1 -> Varying Lowpass Filter/2

== stateflow chart Integration_HILS_Filtered/Subsystem/ModeManageModule/Chart ==
  state ElecMode
    en:
    State=0;
  state OilMode
    en:
    State=1;
  state Exhausted
    en:
    State=2;
  ElecMode -> OilMode [order 1] : [Elec<30]
  (default) -> ElecMode
  OilMode -> ElecMode [order 1] : [Elec>=100 || (Elec>0 && Oil<=0)]
  Exhausted -> ElecMode [order 1] : [Elec>=100 || (Elec>0&&Oil<=0)]
  ElecMode -> Exhausted [order 2] : [Elec<=0 && Oil<=0]
  OilMode -> Exhausted [order 2] : [Elec<=0 && Oil<=0]
  Exhausted -> OilMode [order 2] : [Oil>0]
  data: Elec input; State output; Oil input

== stateflow chart Integration_HILS_Filtered/Subsystem/LedManagementModule/BatteryDisplayModule/Chart3 ==
  state Low
    en:
    du:
    State=1;
  state Adequate1
    en:
    du:
    State=2;
  state Adequate2
    en:
    du:
    State=3;
  state Full
    en,du:
    State=4;
  Adequate1 -> Adequate2 [order 2] : [Battery>30]
  Low -> Adequate1 : [Battery >15]
  Adequate2 -> Adequate1 [order 1] : [Battery<=30]
  Adequate1 -> Low [order 1] : [Battery<=15]
  Full -> Adequate2 : [Battery<=70]
  Adequate2 -> Full [order 2] : [Battery>71]
  (default) -> Full
  data: Battery input; State output

== stateflow chart Integration_HILS_Filtered/Subsystem/LedManagementModule/OilDisplayModule/Chart3 ==
  state Low
    en:
    du:
    State=1;
  state Adequate1
    en:
    du:
    State=2;
  state Adequate2
    en:
    du:
    State=3;
  state Full
    en,du:
    State=4;
  Adequate1 -> Adequate2 [order 2] : [Oil>30]
  Low -> Adequate1 : [Oil >15]
  Adequate2 -> Adequate1 [order 1] : [Oil<=30]
  Adequate1 -> Low [order 1] : [Oil<=15]
  Full -> Adequate2 : [Oil<=70]
  Adequate2 -> Full [order 2] : [Oil>70]
  (default) -> Full
  data: Oil input; State output

== stateflow chart Integration_HILS_Filtered/Subsystem/OilManagement/Chart ==
  state fullOil
    en,du:doubleOil=100;
  state usingOil
    en:
    doubleOil = doubleOil - uint8OilMotorPwm*oilUseRate;
  state chargingOil
    en:
    doubleOil = doubleOil + oilChargeRate;
    doubleOil = doubleOil - uint8OilMotorPwm*oilUseRate;
  state initOil
    en : doubleOil = 100;
  state zeroOil
    en,du: doubleOil =0;
  chargingOil -> fullOil [order 4] : [doubleOil+oilChargeRate-  uint8OilMotorPwm*oilUseRate >= 100]
  fullOil -> usingOil : [uint8OilMotorPwm > 0 && booleanSw1 ==0]
  (default) -> initOil
  chargingOil -> usingOil [order 2] : [booleanSw1 == 0]
  initOil -> usingOil : [uint8OilMotorPwm > 0]
  usingOil -> chargingOil [order 1] : [booleanSw1 == 1]
  usingOil -> usingOil [order 2] : [after(oilUpdateTime,sec)]
  chargingOil -> chargingOil [order 1] : [after(oilUpdateTime,sec)]
  usingOil -> zeroOil [order 3] : [doubleOil - uint8OilMotorPwm*oilUseRate <= 0 ]
  chargingOil -> zeroOil [order 3] : [doubleOil - uint8OilMotorPwm*oilUseRate + oilChargeRate<= 0]
  zeroOil -> chargingOil : [booleanSw1 == 1]
  data: uint8OilMotorPwm input double size=1; booleanSw1 input boolean size=1; doubleOil output double; oilUseRate parameter; oilChargeRate parameter; oilUpdateTime parameter

== stateflow chart Integration_HILS_Filtered/Subsystem/BatteryManagement/Chart ==
  state fullBattery
    en,du:uint8Battery=100;
  state chargingBattery
    en:
    uint8Battery = uint8Battery + (uint16OilMotorSpd*batteryChargeRate)
  state usingBattery
    en:
    uint8Battery=uint8Battery-uint8ElecPwm*batteryUseRate;
  state initBattery
    en : uint8Battery = 100;
  state zeroBattery
    en,du: uint8Battery =0;
  chargingBattery -> fullBattery [order 4] : [uint8Battery+uint16OilMotorSpd*batteryChargeRate >= 100]
  fullBattery -> usingBattery : [uint8ElecPwm > 0 && uint16OilMotorSpd <=0]
  (default) -> initBattery
  chargingBattery -> usingBattery [order 2] : [uint16OilMotorSpd <= 0]
  initBattery -> usingBattery : [uint8ElecPwm > 0]
  usingBattery -> chargingBattery [order 1] : [uint16OilMotorSpd >0]
  chargingBattery -> chargingBattery [order 1] : [after(batteryUpdateTime,sec)]
  usingBattery -> usingBattery [order 2] : [after(batteryUpdateTime,sec)]
  chargingBattery -> zeroBattery [order 3] : [uint8Battery - uint8ElecPwm*batteryUseRate <= 0]
  zeroBattery -> chargingBattery : [uint16OilMotorSpd >0]
  usingBattery -> zeroBattery [order 3] : [uint8Battery - uint8ElecPwm*batteryUseRate <= 0]
  data: uint8ElecPwm input; uint16OilMotorSpd input; uint8Battery output; batteryUpdateTime parameter; batteryUseRate parameter; batteryChargeRate parameter
